simulink model "Song_et_al"  (R2021b)
settings: Solver=VariableStepAuto  StartTime=0.0  StopTime=60  RelTol=1e-10  AbsTol=1e-14
values from neighbouring files (symbols this model uses):
  q0 = [-0.8;0;pi]    [SIM01.m]    (also in SIM02.m = [j 0 the(k)]'; SIM03.m = [-1;0;-pi/2]; SIM04.m = [1 1 k]'; SIM05.m = [2;1;2])
  qr0 = [3;2;1]    [SIM05.m]
settings Model: Creator=PC  LastModifiedBy=PC
settings DataIOCC: SaveFormat=Array

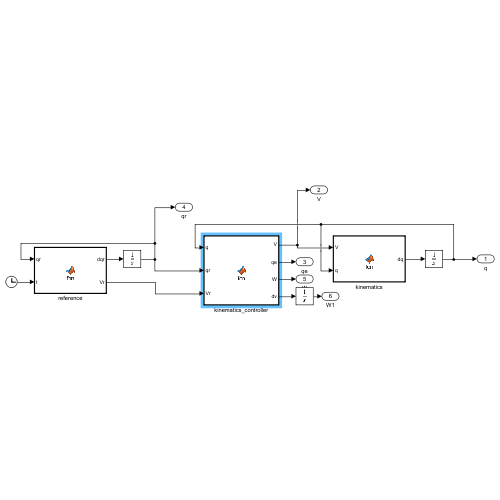
[thumbnail: Simulink's stored preview of the top-level diagram]
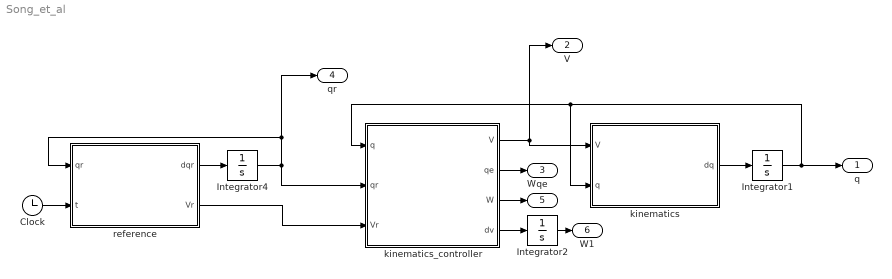
== system Song_et_al ==
  Clock : Clock
  Integrator1 : Integrator  InitialCondition=q0
  Integrator2 : Integrator
  Integrator4 : Integrator  InitialCondition=qr0
  kinematics : MATLAB Function  TreatAsAtomicUnit=on
  kinematics_controller : MATLAB Function  TreatAsAtomicUnit=on
  reference : MATLAB Function  TreatAsAtomicUnit=on
  q : Outport
  V : Outport  Port=2
  qe : Outport  Port=3
  qr : Outport  Port=4
  W : Outport  Port=5
  W1 : Outport  Port=6
  wires:
  Clock/1 -> reference/2(t)
  kinematics_controller/1(V) -> V/1, kinematics/1(V)
  reference/1(dqr) -> Integrator4/1
  Integrator4/1 -> qr/1, reference/1(qr), kinematics_controller/2(qr)
  reference/2(Vr) -> kinematics_controller/3(Vr)
  kinematics_controller/2(qe) -> qe/1
  kinematics/1(dq) -> Integrator1/1
  Integrator1/1 -> kinematics/2(q), kinematics_controller/1(q), q/1
  kinematics_controller/3(W) -> W/1
  kinematics_controller/4(dv) -> Integrator2/1
  Integrator2/1 -> W1/1

== matlab function Song_et_al/reference ==
  data: dqr output size=3*1; qr input size=3*1; Vr output size=2*1; t input
function [dqr,Vr]= fcn(qr,t)
d=0;
vr=0.2;
wr=-atan(0.2*sin(0.2*t));
Vr=[vr;wr];
dqr=[cos(qr(3)) -d*sin(qr(3))
     sin(qr(3))  d*cos(qr(3))
      0          1]*Vr;

== matlab function Song_et_al/kinematics_controller ==
  data: q input size=3*1; V output size=2*1; qr input; Vr input; qe output size=3*1; W output size=2*1; dv output size=1
function [V,qe,W,dv]= fcn(q,qr,Vr)

d=0;
a=0.05;
b=0.28;



vr=Vr(1);
wr=Vr(2);
qe=[ cos(q(3)) sin(q(3)) 0
    -sin(q(3)) cos(q(3)) 0
      0         0        1]*(qr-q);
psi=qe(1)+d*(1-cos(qe(3)));
fi=qe(2)-d*sin(qe(3));

k1=0.25;k2=0.7;k3=0.7;

w1=(vr*cos(qe(3))+k1*tanh(psi))/a + (wr+k2*vr*fi*sin(qe(3))/((1+psi^2+fi^2)*qe(3))+k3*tanh(qe(3)))*b/(2*a);
w2=(vr*cos(qe(3))+k1*tanh(psi))/a - (wr+k2*vr*fi*sin(qe(3))/((1+psi^2+fi^2)*qe(3))+k3*tanh(qe(3)))*b/(2*a);

V=[a/2 a/2;a/b -a/b]*[w1;w2];
W=[w1;w2];
dv=abs(V(1)-vr);

== matlab function Song_et_al/kinematics ==
  data: V input size=2*1; dq output size=3*1; q input size=3*1
function dq = fcn(V,q)
d=0;
dq=[ cos(q(3))  -d*sin(q(3))
     sin(q(3))   d*cos(q(3))
      0          1]*V;
